simulink model "tank_sim"  (R2023b)
settings: Solver=FixedStepAuto  StartTime=0.0  StopTime=10  FixedStep=0.01  RelTol=1e-3
libraries: simulink x3
settings Model: Creator=tomdi  LastModifiedBy=tomdi

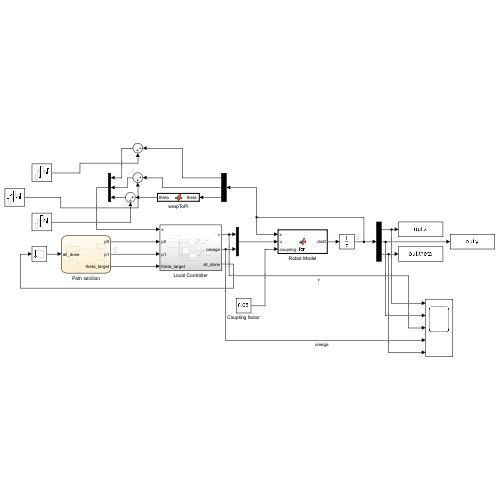
[thumbnail: Simulink's stored preview of the top-level diagram]
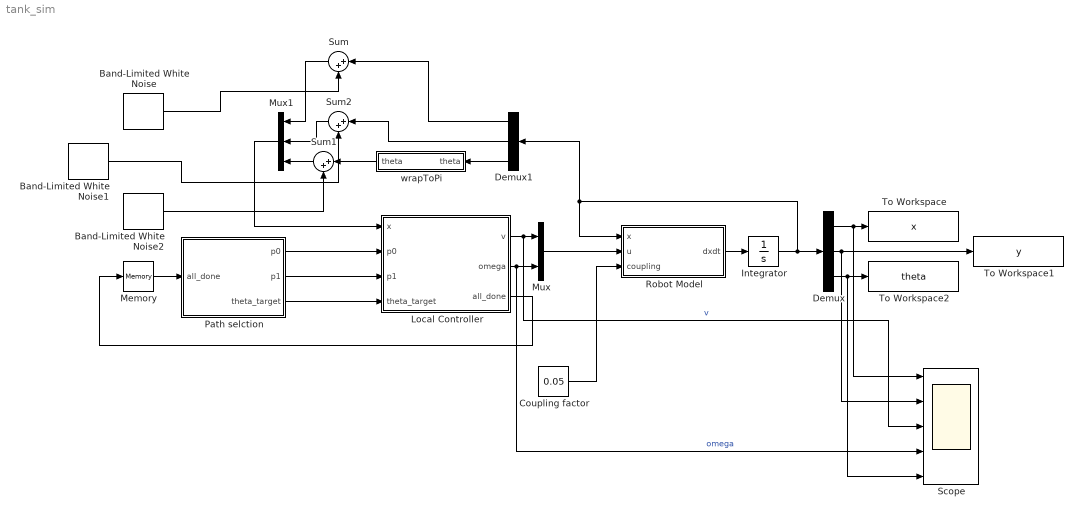
== system tank_sim ==
  Band-Limited White Noise : simulink/Sources/Band-Limited White Noise  Cov=[0.005^2/100]  Ts=0.01  seed=[23341]
  Band-Limited White Noise1 : simulink/Sources/Band-Limited White Noise  Cov=[0.005^2/100]  Ts=0.01  seed=[23341]
  Band-Limited White Noise2 : simulink/Sources/Band-Limited White Noise  Cov=[0.1^2/100]  Ts=0.01  seed=[23341]
  Coupling factor : Constant  Value=0.05
  Demux : Demux  Outputs=3
  Demux1 : Demux  Outputs=3
  Integrator : Integrator  InitialCondition=[0; 0;0]
  Local Controller : Subsystem
  Memory : Memory
  Mux : Mux  Inputs=2
  Mux1 : Mux  Inputs=3
  Path selction : Stateflow chart  TreatAsAtomicUnit=on
      settings: PortSchema="{\"entries\":[{\"content\":{\"sides\":[{\"content\":{\"connectorIds\":[\"In1\"]},\"type\":\"ConnectorPlacement.EquallySpacedRectSide\",\"uuid\":\"5bd98bea-8ff3-4304-985e-ce54fdd492d4\"},{\"content\":{\"connectorIds\":[\"Out2\",\"Out1\",\"Out3\"],\"side\":\"RIGHT\"},\"type\":\"ConnectorPlacement.EquallySpacedRectSide\",\"uuid\":\"0bee52fa-d5bb-4c3f-8969-d01769de831b\"},{\"content\":{\"side\":\"TOP\"},\"type\":\"ConnectorPlacement.EquallySpacedRectSide\",\"uuid\":\"2f6bfcb9-425c-4115-b31c-15d5e2abd278\"}]},\"type\":\"ConnectorPlacement.EquallySpacedConnector\",\"uuid\":\"edcc0c20-79aa-4298-a5a2-b1b335f6c1fb\"}],\"packageUris\":[\"http://schema.mathworks.com/mf0/Connector/R2020b\"],\"version\":\"1.0\"}"
  Robot Model : MATLAB Function  TreatAsAtomicUnit=on
  Scope : Scope  NumInputPorts=5
  Sum : Sum  Inputs=|++
  Sum1 : Sum  Inputs=|++
  Sum2 : Sum  Inputs=|++
  To Workspace : ToWorkspace  VariableName=x  SaveFormat=Timeseries  SampleTime=-1
  To Workspace1 : ToWorkspace  VariableName=y  SaveFormat=Timeseries  SampleTime=-1
  To Workspace2 : ToWorkspace  VariableName=theta  SaveFormat=Timeseries  SampleTime=-1
  wrapToPi : MATLAB Function  TreatAsAtomicUnit=on
  wires:
  Integrator/1 -> Demux/1, Demux1/1, Robot Model/1(x)
  Demux/1 -> Scope/1, To Workspace/1
  Demux/2 -> Scope/2, To Workspace1/1
  Mux/1 -> Robot Model/2(u)
  Robot Model/1(dxdt) -> Integrator/1
  Coupling factor/1 -> Robot Model/3(coupling)
  Local Controller/1(v) -> Scope/3, Mux/1  "v"
  Local Controller/2(omega) -> Scope/4, Mux/2  "omega"
  Path selction/2(p0) -> Local Controller/2(p0)
  Path selction/1(p1) -> Local Controller/3(p1)
  Path selction/3(theta_target) -> Local Controller/4(theta_target)
  Local Controller/3(all_done) -> Memory/1
  Memory/1 -> Path selction/1(all_done)
  Demux/3 -> Scope/5, To Workspace2/1
  wrapToPi/1(theta) -> Sum1/1
  Demux1/3 -> wrapToPi/1("theta ")
  Demux1/2 -> Sum2/1
  Demux1/1 -> Sum/1
  Sum/1 -> Mux1/1
  Sum1/1 -> Mux1/3
  Sum2/1 -> Mux1/2
  Band-Limited White Noise2/1 -> Sum1/2
  Band-Limited White Noise/1 -> Sum/2
  Band-Limited White Noise1/1 -> Sum2/2
  Mux1/1 -> Local Controller/1(x)

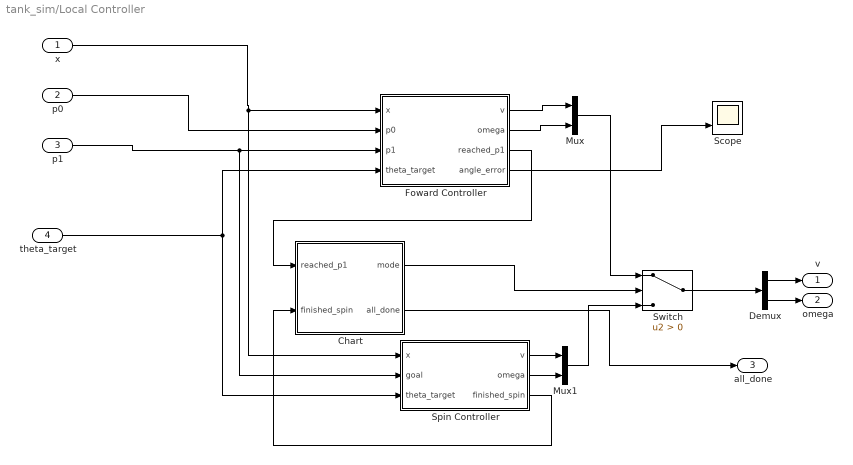
== system tank_sim/Local Controller ==
  x : Inport
  p0 : Inport  Port=2
  p1 : Inport  Port=3
  theta_target : Inport  Port=4
  Chart : Stateflow chart  TreatAsAtomicUnit=on
      settings: PortSchema="{\"entries\":[{\"content\":{\"sides\":[{\"content\":{\"connectorIds\":[\"In2\",\"In1\"]},\"type\":\"ConnectorPlacement.EquallySpacedRectSide\",\"uuid\":\"f679aa5a-5850-4cde-8bb0-53cc0bef3fe8\"},{\"content\":{\"connectorIds\":[\"Out1\",\"Out2\"],\"side\":\"RIGHT\"},\"type\":\"ConnectorPlacement.EquallySpacedRectSide\",\"uuid\":\"53708514-4280-4e39-9668-5ac223c8799a\"},{\"content\":{\"side\":\"TOP\"},\"type\":\"ConnectorPlacement.EquallySpacedRectSide\",\"uuid\":\"3677c3ef-cf04-4c1f-ba74-e9d924f8e91d\"}]},\"type\":\"ConnectorPlacement.EquallySpacedConnector\",\"uuid\":\"55d939be-74bd-4d0f-97de-af99900480d8\"}],\"packageUris\":[\"http://schema.mathworks.com/mf0/Connector/R2020b\"],\"version\":\"1.0\"}"
  Demux : Demux  Outputs=2
  Foward Controller : MATLAB Function  TreatAsAtomicUnit=on
  Mux : Mux  Inputs=2
  Mux1 : Mux  Inputs=2
  Scope : Scope  NumInputPorts=2
  Spin Controller : MATLAB Function  TreatAsAtomicUnit=on
  Switch : Switch  Criteria=u2 > Threshold  SaturateOnIntegerOverflow=off  InputSameDT=off
  v : Outport
  omega : Outport  Port=2
  all_done : Outport  Port=3
  wires:
  p1/1 -> Spin Controller/2(goal), Foward Controller/3(p1)
  Foward Controller/1(v) -> Mux/1
  theta_target/1 -> Spin Controller/3(theta_target), Foward Controller/4(theta_target)
  x/1 -> Spin Controller/1(x), Foward Controller/1(x)
  p0/1 -> Foward Controller/2(p0)
  Foward Controller/2(omega) -> Mux/2
  Foward Controller/3(reached_p1) -> Chart/2(reached_p1)
  Chart/1(mode) -> Switch/2
  Mux/1 -> Switch/1
  Spin Controller/1(v) -> Mux1/1
  Spin Controller/2(omega) -> Mux1/2
  Mux1/1 -> Switch/3
  Spin Controller/3(finished_spin) -> Chart/1(finished_spin)
  Demux/1 -> v/1
  Demux/2 -> omega/1
  Chart/2(all_done) -> all_done/1
  Switch/1 -> Demux/1
  Foward Controller/4(angle_error) -> Scope/2

== matlab function tank_sim/Local Controller/Foward Controller ==
  data: x input; v output size=1; omega output size=1; p0 input; p1 input; reached_p1 output size=1; theta_target input; angle_error output
function [v, omega, reached_p1, angle_error] = fcn(x, p0, p1, theta_target)
    %kax = 0;
    kaa = 5;
    w = 0.5;
    kv = 1;

    theta = x(3);
    r = [x(1); x(2)]; % robot position
    d = p1 - p0;
    k = 1/norm(d)^2 * d' * (r - p0);
    % b = r - k*v - p0;
    % x_p = 1/norm(v) * (b(1)*v(2) - b(2)*v(1));
    s = k*d + p0;
    W = s + w*(p1 - s);

    r_to_waypoint = W - r;
    % try not using atan2 to avoid angle wrapping
    % so measure angle error with a vector
    wr_hat = r_to_waypoint / norm(r_to_waypoint);
    heading = [cos(theta); sin(theta)];
    % this uses the cross product k = ax*by-ay*bx = |a|*|b|*sin(theta)
    % to calculate the actual angle error in a way that doesn't wrap
    sin_angle_error = (heading(1)*wr_hat(2) - heading(2)*wr_hat(1)); % both unit vectors
    cos_angle_error = heading' * wr_hat;
    %desired_angle = atan2(r_to_waypoint(2), r_to_waypoint(1));
    %angle_error = desired_angle - theta;
    angle_error = atan2(sin_angle_error, cos_angle_error);
    % angle_error = asin(sin_angle_error);
    omega = kaa * angle_error;

    % but what if we should be going backwards?
    other_possibility = -wrapToPi(pi - angle_error); % negative since this direction is opposite
    % % angle_error = min(angle_error, other_possibility);
    if abs(angle_error) > abs(other_possibility)
        angle_error = other_possibility;
    end
    omega = kaa * angle_error;

    v = kv * wr_hat' * heading; % handles reversing

    % % if angle is very wrong, correct this first
    % % or, if very near the goal, don't bother moving fowards
    % if abs(angle_error) > pi/6
    %     v = 0; % potential for chatter here
    % end
    reached_p1 = 0;
    if norm(r - p1) < 0.01 % should be smaller so theres room for angular correction to mess things up later
           % should make this 0.01 a parameter
        reached_p1 = 1;
        v = 0;
        omega = 0; % different controller will handle final spin
    end
end

== matlab function tank_sim/Robot Model ==
  data: x input; u input; dxdt output; coupling input
function dxdt = fcn(x,u,coupling)
v = u(1);
omega = u(2);
theta = x(3);
omega = omega + coupling*v;
v = v + coupling*omega;
x_dot = v * cos(theta);
y_dot = v * sin(theta);
theta_dot = omega;
dxdt = [x_dot; y_dot; theta_dot];

== stateflow chart tank_sim/Path selction ==
  state Leg2
    p0 = [1; 0]
    p1 = [1; 1]
    theta_target = pi
  state Leg1
    p0 = [0;0]
    p1 = [1; 0]
    theta_target = -pi/2
  state Leg4
    p0 = [0; 1]
    p1 = [0; 0]
    theta_target = 0
  state Leg3
    p0 = [1; 1]
    p1 = [0; 1]
    theta_target = -pi/2
  (default) -> Leg1
  Leg1 -> Leg2 : [all_done==1]
  Leg2 -> Leg3 : [all_done==1]
  Leg4 -> Leg1 : [all_done==1]
  Leg3 -> Leg4 : [all_done==1]
  data: p1 output; p0 output; theta_target output; all_done input

== stateflow chart tank_sim/Local Controller/Chart ==
  state Forward
    mode = 1;
    all_done = 0;
  state FinalSpin
    mode = 0;
    all_done=0;
  state RequestNext
    all_done=1;
    mode = 0;
  (default) -> Forward
  Forward -> FinalSpin : [reached_p1==1]
  FinalSpin -> RequestNext : [finished_spin==1]
  RequestNext -> Forward
  data: mode output; finished_spin input; reached_p1 input; all_done output

== matlab function tank_sim/Local Controller/Spin Controller ==
  data: x input; goal input; v output size=1; omega output size=1; finished_spin output; theta_target input
function [v, omega, finished_spin] = fcn(x, goal, theta_target)
    kaa = 5;
    kv = 0.2; % making this number too big does kill stuff
    theta = x(3);
    
    r = [x(1); x(2)];
    wr_hat = [cos(theta_target); sin(theta_target)];
    heading = [cos(theta); sin(theta)];
    % this uses the cross product k = ax*by-ay*bx = |a|*|b|*sin(theta)
    % to calculate the actual angle error in a way
    % that doesn't wrap
    sin_angle_error = (heading(1)*wr_hat(2) - heading(2)*wr_hat(1)); % both unit vectors
    %desired_angle = atan2(r_to_waypoint(2), r_to_waypoint(1));
    %angle_error = desired_angle - theta;
    angle_error = asin(sin_angle_error);
    omega = kaa * angle_error;

    % try to keep close to origin
    % control v proportional to it's usefulness
    rg = goal - r;
    rg = rg / norm(rg); % unit vector

    v = kv * rg' * heading;

    finished_spin = 0;
    if abs(angle_error) < 0.01
        finished_spin = 1;
    end
end

== matlab function tank_sim/wrapToPi ==
  data: theta input; theta output
function theta = fcn(theta)

theta = wrapToPi(theta);
